simulink model "HighFiedelity_Simulation"  (R2021b)
settings: Solver=ode45  StartTime=0  StopTime=Stop_Time  FixedStep=Simstep  MaxStep=Simstep  RelTol=1e-5  EnableMultiTasking=on
values from neighbouring files (symbols this model uses):
  Angle_idx = linspace(0,Angle_max,Angle_step)    [A_ToyotaPrius_Flux_Model_Parameter.m]    (also in B1_IPMSM_Machine_Parameter_Init.m)
  Angle_idx_initial = (length(Angle_idx)+1)/2    [A_ToyotaPrius_Flux_Model_Parameter.m]    (also in B1_IPMSM_Machine_Parameter_Init.m)
  flux_d_idx = ParamFluxDIndex    [A_ToyotaPrius_Flux_Model_Parameter.m]    (also in B1_IPMSM_Machine_Parameter_Init.m)
  flux_q_idx = ParamFluxQIndex    [A_ToyotaPrius_Flux_Model_Parameter.m]    (also in B1_IPMSM_Machine_Parameter_Init.m)
  FluxD_Id_Iq_Theta = reshape(Flux_d,Angle_step,I_step,I_step)    [A_ToyotaPrius_Flux_Model_Parameter.m]    (also in B1_IPMSM_Machine_Parameter_Init.m)
  FluxQ_Id_Iq_Theta = reshape(Flux_q,Angle_step,I_step,I_step)    [A_ToyotaPrius_Flux_Model_Parameter.m]    (also in B1_IPMSM_Machine_Parameter_Init.m)
  I_step = 21    [A_ToyotaPrius_Flux_Model_Parameter.m]    (also in B1_IPMSM_Machine_Parameter_Init.m)
  Id_idx = linspace(I_min,I_max,I_step)    [A_ToyotaPrius_Flux_Model_Parameter.m]    (also in B1_IPMSM_Machine_Parameter_Init.m)
  Iq_idx = linspace(I_min,I_max,I_step)    [A_ToyotaPrius_Flux_Model_Parameter.m]    (also in B1_IPMSM_Machine_Parameter_Init.m)
  Step_Time = [0 1 2 3 4 5]    [A0_HighFidelitySimulation.m]    (also in B_PMSM.m = [0.25 0.5 0.75 1])
  Te_Ref_Set = [0.0001 0.00001 0.2 0.3 0.4 0.5]*Motor1.Te_Rated    [A0_HighFidelitySimulation.m]    (also in B_PMSM.m = ones(1,5)*Te_Rated*1)
  Te_SlewRate = inf    [A0_HighFidelitySimulation.m]    (also in B_PMSM.m)
  Torque_Id_Iq_Theta = reshape(Torque_e,Angle_step,I_step,I_step)    [A_ToyotaPrius_Flux_Model_Parameter.m]    (also in B1_IPMSM_Machine_Parameter_Init.m)
  TrqIdmap = ATICALParameterList.Table3D(1).ZAxis    [A_ToyotaPrius_Flux_Model_Parameter.m]    (also in C1_INV1_GainSetting.m)
  TrqIqmap = ATICALParameterList.Table3D(2).ZAxis    [A_ToyotaPrius_Flux_Model_Parameter.m]    (also in C1_INV1_GainSetting.m)
  TrqTId = ATICALParameterList.Table3D(1).YAxis    [A_ToyotaPrius_Flux_Model_Parameter.m]    (also in C1_INV1_GainSetting.m)
  TrqTIq = ATICALParameterList.Table3D(2).YAxis    [A_ToyotaPrius_Flux_Model_Parameter.m]    (also in C1_INV1_GainSetting.m)
  TrqWrId = ATICALParameterList.Table3D(1).XAxis    [A_ToyotaPrius_Flux_Model_Parameter.m]    (also in C1_INV1_GainSetting.m)
  TrqWrIq = ATICALParameterList.Table3D(2).XAxis    [A_ToyotaPrius_Flux_Model_Parameter.m]    (also in C1_INV1_GainSetting.m)
  Vdc = 650    [A0_HighFidelitySimulation.m]    (also in B_PMSM.m)
  Wrpm_Ref_Set = [5000 5000 5000 5000 5000]    [A0_HighFidelitySimulation.m]    (also in B_PMSM.m = Wrm_Init*ones(1,5))
undefined symbols (not defined in the file or in its folder): DCMotor, DiscIntNeverNeededParam, idmap, INV1, INV2, iqmap, Motor1
libraries: simulink x3
settings Model: SimulationMode=accelerator  Creator=KYC  LastModifiedBy=jun
settings SolverCC: AlgebraicLoopSolver=TrustRegion
settings DataIOCC: LimitDataPoints=on  SaveFormat=Array  ReturnWorkspaceOutputs=off
settings OptimizationCC: LifeSpan=inf
settings DebuggingCC: UnderspecifiedInitializationDetection=Classic  MergeDetectMultiDrivingBlocksExec=none  SolverPrmCheckMsg=warning  InheritedTsInSrcMsg=none  AllowSymbolicDim=off  StateNameClashWarn=warning  SFUnexpectedBacktrackingDiag=warning  SFNoUnconditionalDefaultTransitionDiag=warning  SFExecutionAtInitializationDiag=none  SFMachineParentedDataDiag=warning  ArithmeticOperatorsInVariantConditions=warning
settings HardwareCC: ProdBitPerPointer=32  ProdBitPerSizeT=32  ProdBitPerPtrDiffT=32  ProdLargestAtomicFloat=None  ProdIntDivRoundTo=Undefined  ProdEndianess=Unspecified  ProdWordSize=32  ProdHWDeviceType=32-bit Generic
settings ModelReferenceCC: PropagateSignalLabelsOutOfModel=off
settings SFSimCC: SimUseLocalCustomCode=off  CustomCodeUndefinedFunction=UseInterfaceOnly
settings RTWCC: RTWUseLocalCustomCode=off
settings CodeAppCC: StateflowObjectComments=on
settings GRTTargetCC: TargetLangStandard=C89/C90 (ANSI)
settings ConfigComp: CovMetricSettings=dw  CovSaveCumulativeToWorkspaceVar=on  CovSaveSingleToWorkspaceVar=on  CovExternalEMLEnable=off  CovSFcnEnable=off

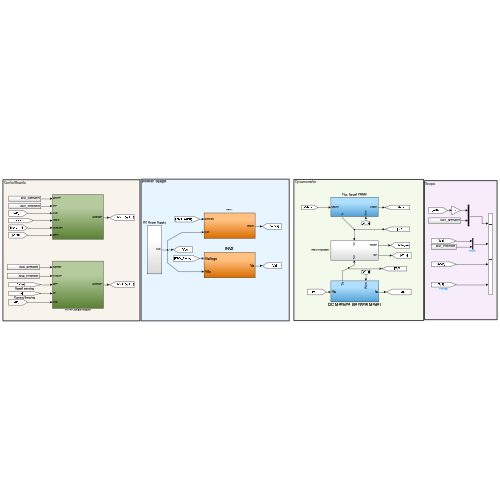
[thumbnail: Simulink's stored preview of the top-level diagram]
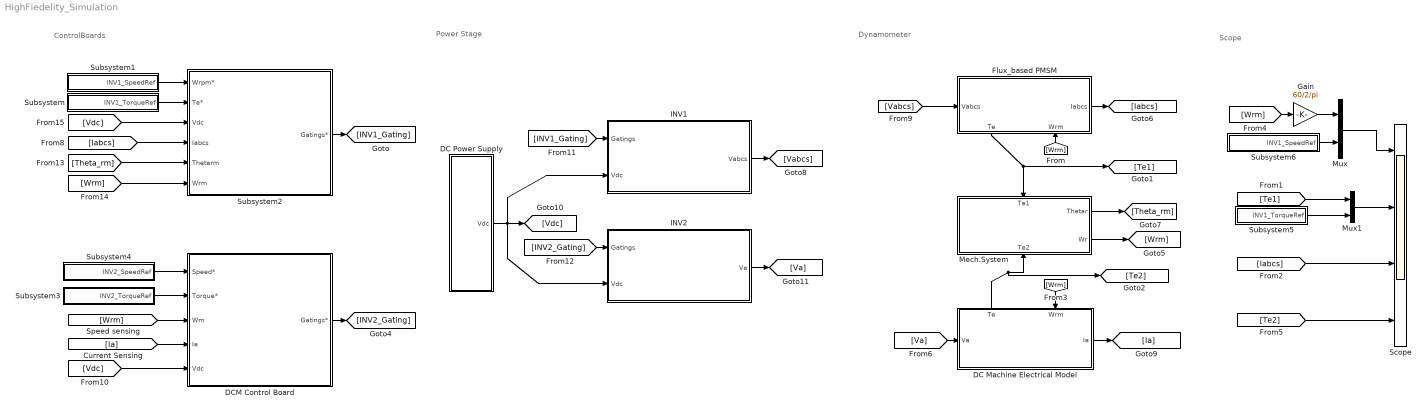
== system HighFiedelity_Simulation ==
  note: Scope
  note: ControlBoards
  note: Dynamometer
  note: Power Stage
  DC Machine Electrical Model : Subsystem
      settings: PortSchema="{\"entries\":[{\"content\":{\"sides\":[{\"content\":{\"connectorIds\":[\"In1\"]},\"type\":\"ConnectorPlacement.EquallySpacedRectSide\",\"uuid\":\"4074897e-6920-4f33-b302-64d86120b7df\"},{\"content\":{\"connectorIds\":[\"Out1\"],\"side\":\"RIGHT\"},\"type\":\"ConnectorPlacement.EquallySpacedRectSide\",\"uuid\":\"671615ca-e362-48c9-a030-03d33faae874\"},{\"content\":{\"connectorIds\":[\"Out2\",\"In2\"],\"side\":\"TOP\"},\"type\":\"ConnectorPlacement.EquallySpacedRectSide\",\"uuid\":\"d587e8fb-b462-47db-b9f9-66f25c83a3fe\"},{\"content\":{\"connectorIds\":[],\"side\":\"BOTTOM\"},\"type\":\"ConnectorPlacement.EquallySpacedRectSide\",\"uuid\":\"9be21003-cb0d-41fd-b790-e70774da76cb\"}]},\"type\":\"ConnectorPlacement.EquallySpacedConnector\",\"uuid\":\"22d4a5b5-b610-40ac-ac45-102e1f1adc00\"}],\"packageUris\":[\"http://schema.mathworks.com/mf0/Connector/R2020b\"],\"version\":\"1.0\"}"
  DC Power Supply : Subsystem
  DCM Control Board : Subsystem
  Flux_based PMSM : Subsystem
      settings: PortSchema="{\"entries\":[{\"content\":{\"sides\":[{\"content\":{\"connectorIds\":[\"In1\"]},\"type\":\"ConnectorPlacement.EquallySpacedRectSide\",\"uuid\":\"24322e7c-2896-443d-bb86-37c4d4149ef5\"},{\"content\":{\"connectorIds\":[\"Out1\"],\"side\":\"RIGHT\"},\"type\":\"ConnectorPlacement.EquallySpacedRectSide\",\"uuid\":\"a5d08852-92bf-4b5a-af83-42822b482983\"},{\"content\":{\"connectorIds\":[],\"side\":\"TOP\"},\"type\":\"ConnectorPlacement.EquallySpacedRectSide\",\"uuid\":\"64930a76-1018-4eab-af8e-9c2112ff20c6\"},{\"content\":{\"connectorIds\":[\"Out2\",\"In2\"],\"side\":\"BOTTOM\"},\"type\":\"ConnectorPlacement.EquallySpacedRectSide\",\"uuid\":\"89450d1c-3f7d-44a3-8810-d67b8ce20cc5\"}]},\"type\":\"ConnectorPlacement.EquallySpacedConnector\",\"uuid\":\"0cf1f8cb-98d5-4acc-99e3-a93106a75429\"}],\"packageUris\":[\"http://schema.mathworks.com/mf0/Connector/R2020b\"],\"version\":\"1.0\"}"
  Gain : Gain  Gain=60/2/pi
  INV1 : Subsystem
  INV2 : Subsystem
  Mech.System : Subsystem
      settings: PortSchema="{\"entries\":[{\"content\":{\"sides\":[{\"content\":{\"connectorIds\":[]},\"type\":\"ConnectorPlacement.EquallySpacedRectSide\",\"uuid\":\"7816393c-e6ef-44df-b641-25156ded1cdc\"},{\"content\":{\"connectorIds\":[\"Out1\",\"Out2\"],\"side\":\"RIGHT\"},\"type\":\"ConnectorPlacement.EquallySpacedRectSide\",\"uuid\":\"df3d9513-253d-4c97-8efd-af2438fb286e\"},{\"content\":{\"connectorIds\":[\"In1\"],\"side\":\"TOP\"},\"type\":\"ConnectorPlacement.EquallySpacedRectSide\",\"uuid\":\"65b6b526-a008-40f6-a42d-b2e1dc0c5f24\"},{\"content\":{\"connectorIds\":[\"In2\"],\"side\":\"BOTTOM\"},\"type\":\"ConnectorPlacement.EquallySpacedRectSide\",\"uuid\":\"f448aff5-19c1-43a0-84ba-52356c379f88\"}]},\"type\":\"ConnectorPlacement.EquallySpacedConnector\",\"uuid\":\"afd6e091-39ce-476c-80f4-568492feeb85\"}],\"packageUris\":[\"http://schema.mathworks.com/mf0/Connector/R2020b\"],\"version\":\"1.0\"}"
  Mux : Mux  Inputs=2
  Mux1 : Mux  Inputs=2
  Scope : Scope  NumInputPorts=4
  Subsystem : Subsystem
  Subsystem1 : Subsystem
  Subsystem2 : Subsystem
  Subsystem3 : Subsystem
  Subsystem4 : Subsystem
  Subsystem5 : Subsystem
  Subsystem6 : Subsystem
  wires:
  Flux_based PMSM/1(Iabcs) -> [Iabcs]
  [Vabcs] -> Flux_based PMSM/1(Vabcs)
  DCM Control Board/1(Gatings*) -> [INV2_Gating]
  [Wrm] -> DCM Control Board/3(Wm)
  [Vdc] -> DCM Control Board/5(Vdc)
  [Ia] -> DCM Control Board/4(Ia)
  Subsystem3/1(INV2_TorqueRef) -> DCM Control Board/2(Torque*)
  Mech.System/2(Wr) -> [Wrm]
  Mech.System/1(Thetar) -> [Theta_rm]
  DC Machine Electrical Model/2(Te) -> [Te2], Mech.System/2(Te2)
  Flux_based PMSM/2(Te) -> [Te1], Mech.System/1(Te1)
  [INV1_Gating] -> INV1/1(Gatings)
  [INV2_Gating] -> INV2/1(Gatings)
  DC Power Supply/1(Vdc) -> INV1/2(Vdc), [Vdc], INV2/2(Vdc)
  INV1/1(Vabcs) -> [Vabcs]
  INV2/1(Va) -> [Va]
  Subsystem2/1(Gatings*) -> [INV1_Gating]
  [Wrm] -> Flux_based PMSM/2(Wrm)
  [Wrm] -> DC Machine Electrical Model/2(Wrm)
  [Va] -> DC Machine Electrical Model/1(Va)
  Subsystem1/1(INV1_SpeedRef) -> Subsystem2/1(Wrpm*)
  Subsystem/1(INV1_TorqueRef) -> Subsystem2/2(Te*)
  [Vdc] -> Subsystem2/3(Vdc)
  [Iabcs] -> Subsystem2/4(Iabcs)
  [Theta_rm] -> Subsystem2/5(Thetarm)
  [Wrm] -> Subsystem2/6(Wrm)
  [Wrm] -> Gain/1
  Gain/1 -> Mux/1
  Subsystem6/1(INV1_SpeedRef) -> Mux/2
  Mux/1 -> Scope/1
  [Iabcs] -> Scope/3
  Subsystem5/1(INV1_TorqueRef) -> Mux1/2
  Mux1/1 -> Scope/2
  [Te1] -> Mux1/1
  DC Machine Electrical Model/1(Ia) -> [Ia]
  Subsystem4/1(INV2_SpeedRef) -> DCM Control Board/1(Speed*)
  [Te2] -> Scope/4

== system HighFiedelity_Simulation/DC Machine Electrical Model ==
  note: DC Machine Electrical Model
  Va : Inport
  Wrm : Inport  Port=2
  1/La2 : Gain  Gain=DCMotor.K  SaturateOnIntegerOverflow=on  OutDataTypeStr=Inherit: Same as input  ParamDataTypeStr=Inherit: Same as input
  Gain2 : Gain  Gain=1/DCMotor.La
  Gain3 : Gain  Gain=DCMotor.Ra
  Gain4 : Gain  Gain=DCMotor.K
  Integrator1 : Integrator
  Sum : Sum  Inputs=+--  SaturateOnIntegerOverflow=on
  Ia : Outport
  Te : Outport  Port=2  VectorParamsAs1DForOutWhenUnconnected=off
  wires:
  1/La2/1 -> Sum/2
  Integrator1/1 -> Gain4/1, Ia/1, Gain3/1
  Sum/1 -> Gain2/1
  Gain4/1 -> Te/1
  Va/1 -> Sum/1
  Gain2/1 -> Integrator1/1
  Gain3/1 -> Sum/3
  Wrm/1 -> 1/La2/1

== system HighFiedelity_Simulation/DC Power Supply ==
  Constant : Constant  Value=Vdc
  Vdc : Outport
  wires:
  Constant/1 -> Vdc/1

== system HighFiedelity_Simulation/DCM Control Board ==
  Speed* : Inport
  Torque* : Inport  Port=2
  Wm : Inport  Port=3
  Ia : Inport  Port=4
  Vdc : Inport  Port=5
  Control Programs : Subsystem
  Fsw : DiscretePulseGenerator  PulseType=Time based  Period=1/INV2.SwitchingFrequency  PulseWidth=50
  Gain : Gain  Gain=-1
  PWM Module : Subsystem
  Gatings* : Outport
  wires:
  PWM Module/1(Gating) -> Gatings*/1
  Speed*/1 -> Control Programs/1(Speed*)
  Torque*/1 -> Control Programs/2(Torque*)
  Wm/1 -> Gain/1
  Ia/1 -> Control Programs/4(Ia)
  Fsw/1 -> Control Programs/Trigger
  Control Programs/1(Counter) -> PWM Module/1(Counter)
  Vdc/1 -> Control Programs/5(Vdc)
  Gain/1 -> Control Programs/3(Wm)

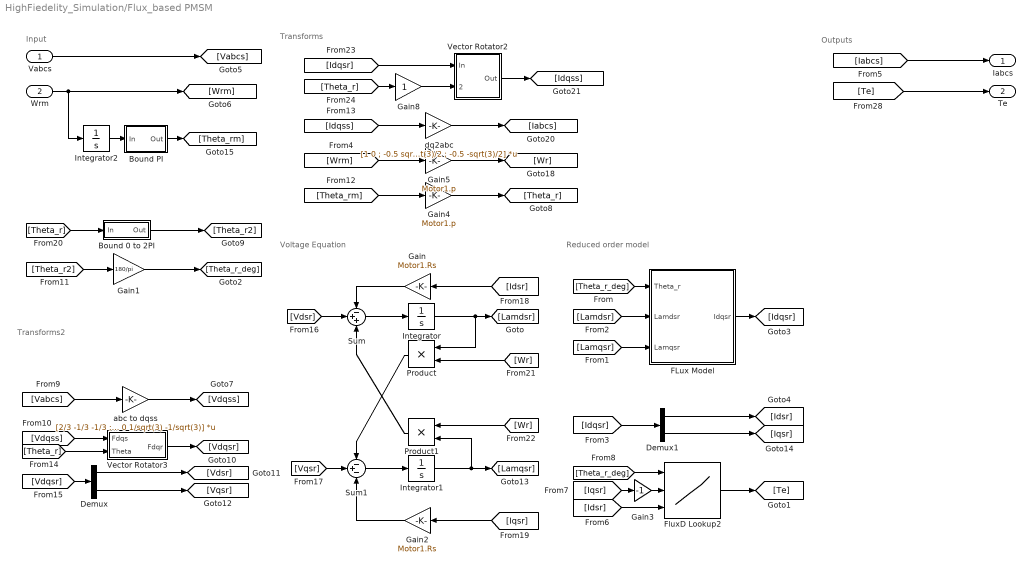
== system HighFiedelity_Simulation/Flux_based PMSM ==
  note: Transforms
  note: Reduced order model
  note: Voltage Equation
  note: Transforms2
  note: Input
  note: Outputs
  Vabcs : Inport
  Wrm : Inport  Port=2
  Bound 0 to 2PI : Subsystem
  Bound PI : Subsystem
  Demux : Demux  Outputs=2
  Demux1 : Demux  Outputs=2
  FLux Model : Subsystem
  FluxD Lookup2 : Lookup_n-D  NumberOfTableDimensions=3  BreakpointsForDimension1=Angle_idx  BreakpointsForDimension2=Id_idx  BreakpointsForDimension3=Iq_idx  Table=Torque_Id_Iq_Theta  InternalRulePriority=Speed  RndMeth=Simplest  InputSameDT=on
      settings: InputPortMap=u0,u1,u2
  Gain : Gain  Gain=Motor1.Rs
  Gain1 : Gain  Gain=180/pi
  Gain2 : Gain  Gain=Motor1.Rs
  Gain3 : Gain  Gain=-1
  Gain4 : Gain  Gain=Motor1.p
  Gain5 : Gain  Gain=Motor1.p
  Gain8 : Gain
  Integrator : Integrator  InitialCondition=FluxD_Id_Iq_Theta(Angle_idx_initial,(I_step+1)/2,(I_step+1)/2)
  Integrator1 : Integrator  InitialCondition=FluxQ_Id_Iq_Theta(Angle_idx_initial,(I_step+1)/2,(I_step+1)/2)
  Integrator2 : Integrator
  Product : Product
  Product1 : Product
  Sum : Sum  Inputs=-++
  Sum1 : Sum  Inputs=-+-
  Vector Rotator2 : Subsystem
  Vector Rotator3 : Subsystem
  abc to dqss : Gain  Gain=[2/3 -1/3 -1/3 ; 0 1/sqrt(3) -1/sqrt(3)]  Multiplication=Matrix(K*u)
  dq2abc : Gain  Gain=[1 0 ; -0.5 sqrt(3)/2 ; -0.5 -sqrt(3)/2]  Multiplication=Matrix(K*u)
  Iabcs : Outport
  Te : Outport  Port=2
  wires:
  [Theta_r] -> Vector Rotator3/2(Theta)
  Vabcs/1 -> [Vabcs]
  [Vdqss] -> Vector Rotator3/1(Fdqs)
  Vector Rotator3/1(Fdqr) -> [Vdqsr]
  [Vabcs] -> abc to dqss/1
  abc to dqss/1 -> [Vdqss]
  Bound 0 to 2PI/1(Out) -> [Theta_r2]
  [Theta_r] -> Bound 0 to 2PI/1(In)
  [Theta_r2] -> Gain1/1
  [Iqsr] -> Gain3/1
  [Idsr] -> FluxD Lookup2/3
  [Theta_r_deg] -> FluxD Lookup2/1
  [Vdqsr] -> Demux/1
  Demux/2 -> [Vqsr]
  Demux/1 -> [Vdsr]
  [Vdsr] -> Sum/2
  [Vqsr] -> Sum1/2
  Gain/1 -> Sum/1
  [Idsr] -> Gain/1
  [Iqsr] -> Gain2/1
  Gain2/1 -> Sum1/3
  Sum/1 -> Integrator/1
  Integrator/1 -> Product/1, [Lamdsr]
  [Wr] -> Product/2
  Product/1 -> Sum1/1
  Sum1/1 -> Integrator1/1
  Integrator1/1 -> Product1/2, [Lamqsr]
  [Wr] -> Product1/1
  Product1/1 -> Sum/3
  [Theta_r_deg] -> FLux Model/1(Theta_r)
  [Lamdsr] -> FLux Model/2(Lamdsr)
  [Lamqsr] -> FLux Model/3(Lamqsr)
  [Idqsr] -> Demux1/1
  Demux1/2 -> [Iqsr]
  Gain1/1 -> [Theta_r_deg]
  Gain3/1 -> FluxD Lookup2/2
  FLux Model/1(Idqsr) -> [Idqsr]
  Gain4/1 -> [Theta_r]
  [Idqss] -> dq2abc/1
  dq2abc/1 -> [Iabcs]
  Gain5/1 -> [Wr]
  [Wrm] -> Gain5/1
  [Theta_rm] -> Gain4/1
  Vector Rotator2/1(Out) -> [Idqss]
  [Theta_r] -> Gain8/1
  Gain8/1 -> Vector Rotator2/2(Theta)
  [Idqsr] -> Vector Rotator2/1(In)
  [Iabcs] -> Iabcs/1
  [Te] -> Te/1
  FluxD Lookup2/1 -> [Te]
  Demux1/1 -> [Idsr]
  Wrm/1 -> Integrator2/1, [Wrm]
  Bound PI/1(Out) -> [Theta_rm]
  Integrator2/1 -> Bound PI/1(In)

== system HighFiedelity_Simulation/INV1 ==
  Gatings : Inport
  Vdc : Inport  Port=2
  Product : Product
  Vabcs : Outport
  wires:
  Gatings/1 -> Product/1
  Vdc/1 -> Product/2
  Product/1 -> Vabcs/1

== system HighFiedelity_Simulation/INV2 ==
  Gatings : Inport
  Vdc : Inport  Port=2
  Product : Product
  Va : Outport  InitialOutput=0  VectorParamsAs1DForOutWhenUnconnected=off
  wires:
  Vdc/1 -> Product/2
  Product/1 -> Va/1
  Gatings/1 -> Product/1

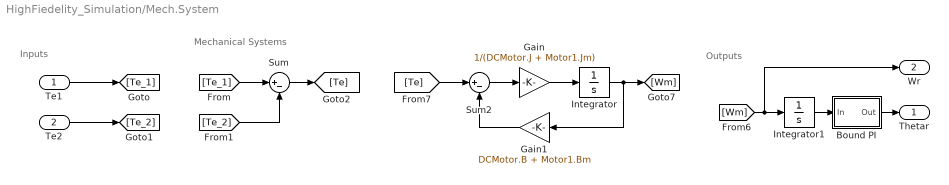
== system HighFiedelity_Simulation/Mech.System ==
  note: Outputs
  note: Mechanical Systems
  note: Inputs
  Te1 : Inport
  Te2 : Inport  Port=2
  Bound PI : Subsystem
  Gain : Gain  Gain=1/(DCMotor.J + Motor1.Jm)
  Gain1 : Gain  Gain=DCMotor.B + Motor1.Bm
  Integrator : Integrator
  Integrator1 : Integrator
  Sum : Sum  Inputs=|+-
  Sum2 : Sum  Inputs=|+-
  Thetar : Outport  VectorParamsAs1DForOutWhenUnconnected=off
  Wr : Outport  Port=2
  wires:
  Sum2/1 -> Gain/1
  Gain1/1 -> Sum2/2
  Gain/1 -> Integrator/1
  Integrator/1 -> Gain1/1, [Wm]
  Te1/1 -> [Te_1]
  Te2/1 -> [Te_2]
  [Te_1] -> Sum/1
  [Te_2] -> Sum/2
  Sum/1 -> [Te]
  [Te] -> Sum2/1
  Bound PI/1(Out) -> Thetar/1
  Integrator1/1 -> Bound PI/1(In)
  [Wm] -> Wr/1, Integrator1/1

== system HighFiedelity_Simulation/Subsystem ==
  Add : Sum  Inputs=++++
  Rate Limiter : RateLimiter  RisingSlewLimit=Te_SlewRate*Motor1.Te_Rated  FallingSlewLimit=-Te_SlewRate*Motor1.Te_Rated  SampleTimeMode=inherited
  Scope : Scope  NumInputPorts=2
  Step1 : Step  Time=Step_Time(1)  Before=Te_Ref_Set(1)  After=Te_Ref_Set(2)
  Step2 : Step  Time=Step_Time(3)  After=Te_Ref_Set(4)-Te_Ref_Set(3)
  Step3 : Step  Time=Step_Time(2)  After=Te_Ref_Set(3)-Te_Ref_Set(2)
  Step4 : Step  Time=Step_Time(4)  After=Te_Ref_Set(5)-Te_Ref_Set(4)
  INV1_TorqueRef : Outport
  wires:
  Step2/1 -> Add/3
  Step4/1 -> Add/4
  Step3/1 -> Add/2
  Step1/1 -> Add/1
  Rate Limiter/1 -> Scope/2, INV1_TorqueRef/1
  Add/1 -> Scope/1, Rate Limiter/1

== system HighFiedelity_Simulation/Subsystem1 ==
  Add : Sum  Inputs=++++
  Step1 : Step  Time=Step_Time(1)  Before=Wrpm_Ref_Set(1)  After=Wrpm_Ref_Set(2)
  Step2 : Step  Time=Step_Time(3)  After=Wrpm_Ref_Set(4)-Wrpm_Ref_Set(3)
  Step3 : Step  Time=Step_Time(2)  After=Wrpm_Ref_Set(3)-Wrpm_Ref_Set(2)
  Step4 : Step  Time=Step_Time(4)  After=Wrpm_Ref_Set(5)-Wrpm_Ref_Set(4)
  INV1_SpeedRef : Outport
  wires:
  Step1/1 -> Add/1
  Step3/1 -> Add/2
  Step4/1 -> Add/4
  Step2/1 -> Add/3
  Add/1 -> INV1_SpeedRef/1

== system HighFiedelity_Simulation/Subsystem2 ==
  Wrpm* : Inport
  Te* : Inport  Port=2
  Vdc : Inport  Port=3
  Iabcs : Inport  Port=4
  Thetarm : Inport  Port=5
  Wrm : Inport  Port=6
  Digital Controller : Subsystem
  PWM Module : Subsystem
  Pulse Generator2 : DiscretePulseGenerator  PulseType=Time based  Period=INV1.Ts  PulseWidth=50
  Gatings* : Outport
  wires:
  Digital Controller/1(Counter) -> PWM Module/1(Counter)
  Iabcs/1 -> Digital Controller/4(Iabcs)
  Te*/1 -> Digital Controller/2(Te*)
  Thetarm/1 -> Digital Controller/5(Thetarm)
  Pulse Generator2/1 -> Digital Controller/Trigger
  Vdc/1 -> Digital Controller/3(Vdc)
  Wrm/1 -> Digital Controller/6(Wrm)
  Wrpm*/1 -> Digital Controller/1(Wrpm*)
  PWM Module/1(Gatings) -> Gatings*/1

== system HighFiedelity_Simulation/Subsystem3 ==
  Add : Sum  Inputs=++++
  Rate Limiter : RateLimiter  RisingSlewLimit=Te_SlewRate*Motor1.Te_Rated  FallingSlewLimit=-Te_SlewRate*Motor1.Te_Rated  SampleTimeMode=inherited
  Step1 : Step  Time=Step_Time(1)  Before=Te_Ref_Set(1)  After=Te_Ref_Set(2)
  Step2 : Step  Time=Step_Time(3)  After=Te_Ref_Set(4)-Te_Ref_Set(3)
  Step3 : Step  Time=Step_Time(2)  After=Te_Ref_Set(3)-Te_Ref_Set(2)
  Step4 : Step  Time=Step_Time(4)  After=Te_Ref_Set(5)-Te_Ref_Set(4)
  INV2_TorqueRef : Outport
  wires:
  Step2/1 -> Add/3
  Step4/1 -> Add/4
  Step3/1 -> Add/2
  Step1/1 -> Add/1
  Rate Limiter/1 -> INV2_TorqueRef/1
  Add/1 -> Rate Limiter/1

== system HighFiedelity_Simulation/Subsystem4 ==
  Add : Sum  Inputs=++++
  Gain : Gain  Gain=-1
  Step1 : Step  Time=Step_Time(1)  Before=Wrpm_Ref_Set(1)  After=Wrpm_Ref_Set(2)
  Step2 : Step  Time=Step_Time(3)  After=Wrpm_Ref_Set(4)-Wrpm_Ref_Set(3)
  Step3 : Step  Time=Step_Time(2)  After=Wrpm_Ref_Set(3)-Wrpm_Ref_Set(2)
  Step4 : Step  Time=Step_Time(4)  After=Wrpm_Ref_Set(5)-Wrpm_Ref_Set(4)
  INV2_SpeedRef : Outport
  wires:
  Step1/1 -> Add/1
  Step3/1 -> Add/2
  Step4/1 -> Add/4
  Step2/1 -> Add/3
  Gain/1 -> INV2_SpeedRef/1
  Add/1 -> Gain/1

== system HighFiedelity_Simulation/Subsystem5 ==
  Add : Sum  Inputs=++++
  Rate Limiter : RateLimiter  RisingSlewLimit=Te_SlewRate*Motor1.Te_Rated  FallingSlewLimit=-Te_SlewRate*Motor1.Te_Rated  SampleTimeMode=inherited
  Step1 : Step  Time=Step_Time(1)  Before=Te_Ref_Set(1)  After=Te_Ref_Set(2)
  Step2 : Step  Time=Step_Time(3)  After=Te_Ref_Set(4)-Te_Ref_Set(3)
  Step3 : Step  Time=Step_Time(2)  After=Te_Ref_Set(3)-Te_Ref_Set(2)
  Step4 : Step  Time=Step_Time(4)  After=Te_Ref_Set(5)-Te_Ref_Set(4)
  INV1_TorqueRef : Outport
  wires:
  Step2/1 -> Add/3
  Step4/1 -> Add/4
  Step3/1 -> Add/2
  Step1/1 -> Add/1
  Rate Limiter/1 -> INV1_TorqueRef/1
  Add/1 -> Rate Limiter/1

== system HighFiedelity_Simulation/Subsystem6 ==
  Add : Sum  Inputs=++++
  Step1 : Step  Time=Step_Time(1)  Before=Wrpm_Ref_Set(1)  After=Wrpm_Ref_Set(2)
  Step2 : Step  Time=Step_Time(3)  After=Wrpm_Ref_Set(4)-Wrpm_Ref_Set(3)
  Step3 : Step  Time=Step_Time(2)  After=Wrpm_Ref_Set(3)-Wrpm_Ref_Set(2)
  Step4 : Step  Time=Step_Time(4)  After=Wrpm_Ref_Set(5)-Wrpm_Ref_Set(4)
  INV1_SpeedRef : Outport
  wires:
  Step1/1 -> Add/1
  Step3/1 -> Add/2
  Step4/1 -> Add/4
  Step2/1 -> Add/3
  Add/1 -> INV1_SpeedRef/1

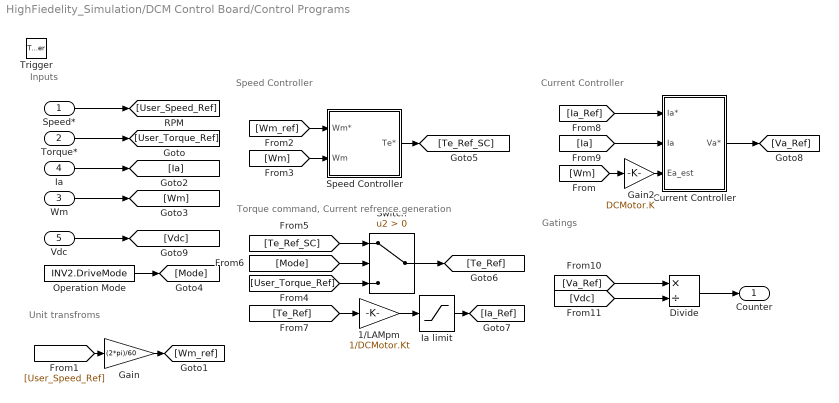
== system HighFiedelity_Simulation/DCM Control Board/Control Programs ==
  note: Speed Controller
  note: Unit transfroms
  note: Inputs
  note: Current Controller
  note: Gatings
  note: Torque command, Current refrence generation
  Speed* : Inport
  Torque* : Inport  Port=2
  Wm : Inport  Port=3
  Ia : Inport  Port=4
  Vdc : Inport  Port=5
  Trigger : TriggerPort  VariantControl=(inherit)  PortDimensions=1
  1/LAMpm : Gain  Gain=1/DCMotor.Kt  SaturateOnIntegerOverflow=on  OutDataTypeStr=Inherit: Same as input  ParamDataTypeStr=Inherit: Same as input
  Current Controller : Subsystem
  Divide : Product  Inputs=*/
  Gain : Gain  Gain=(2*pi)/60
  Gain2 : Gain  Gain=DCMotor.K
  Ia limit : Saturate  UpperLimit=DCMotor.Ia_limit  LowerLimit=-DCMotor.Ia_limit
  Operation Mode : Constant  Value=INV2.DriveMode
  Speed Controller : Subsystem
  Switch : Switch  Criteria=u2 > Threshold
  Counter : Outport
  wires:
  Speed*/1 -> [User_Speed_Ref]
  Gain/1 -> [Wm_ref]
  Gain2/1 -> Current Controller/3(Ea_est)
  Torque*/1 -> [User_Torque_Ref]
  [Te_Ref] -> 1/LAMpm/1
  Speed Controller/1(Te*) -> [Te_Ref_SC]
  Ia/1 -> [Ia]
  [Ia_Ref] -> Current Controller/1(Ia*)
  Switch/1 -> [Te_Ref]
  [Ia] -> Current Controller/2(Ia)
  [Mode] -> Switch/2
  Ia limit/1 -> [Ia_Ref]
  Operation Mode/1 -> [Mode]
  [User_Torque_Ref] -> Switch/3
  [Wm] -> Gain2/1
  1/LAMpm/1 -> Ia limit/1
  [User_Speed_Ref] -> Gain/1
  [Te_Ref_SC] -> Switch/1
  [Wm] -> Speed Controller/2(Wm)
  [Wm_ref] -> Speed Controller/1(Wm*)
  Wm/1 -> [Wm]
  Vdc/1 -> [Vdc]
  [Va_Ref] -> Divide/1
  Divide/1 -> Counter/1
  [Vdc] -> Divide/2
  Current Controller/1(Va*) -> [Va_Ref]

== system HighFiedelity_Simulation/DCM Control Board/PWM Module ==
  Counter : Inport
  Carrier wave : simulink/Sources/Repeating Sequence  rep_seq_t="[0  1/2/INV2.SwitchingFrequency  1/INV2.SwitchingFrequency]"  rep_seq_y=[-1 1 -1]
  Sum2 : Sum  Inputs=+-  SaturateOnIntegerOverflow=on
  Gating : Outport
  wires:
  Counter/1 -> Sum2/1
  Carrier wave/1 -> Sum2/2
  Sum2/1 -> Gating/1

== system HighFiedelity_Simulation/Flux_based PMSM/Bound 0 to 2PI ==
  In : Inport
  Fcn1 : Fcn  Expr=1/(2*pi)*u+0.5
  Fcn2 : Fcn  Expr=u-floor(u)
  Fcn3 : Fcn  Expr=2*pi*(u)
  Out : Outport
  wires:
  Fcn1/1 -> Fcn2/1
  Fcn2/1 -> Fcn3/1
  In/1 -> Fcn1/1
  Fcn3/1 -> Out/1

== system HighFiedelity_Simulation/Flux_based PMSM/Bound PI ==
  In : Inport
  Fcn1 : Fcn  Expr=1/(2*pi)*u+0.5
  Fcn2 : Fcn  Expr=u-floor(u)
  Fcn3 : Fcn  Expr=2*pi*(u-0.5)
  Out : Outport
  wires:
  Fcn1/1 -> Fcn2/1
  Fcn2/1 -> Fcn3/1
  In/1 -> Fcn1/1
  Fcn3/1 -> Out/1

== system HighFiedelity_Simulation/Flux_based PMSM/FLux Model ==
  Theta_r : Inport
  Lamdsr : Inport  Port=2
  Lamqsr : Inport  Port=3
  IC : InitialCondition  Value=0
  IC1 : InitialCondition  Value=0
  Id Lookup : Lookup_n-D  NumberOfTableDimensions=3  BreakpointsForDimension1=Angle_idx  BreakpointsForDimension2=flux_d_idx  BreakpointsForDimension3=flux_q_idx  Table=idmap  InternalRulePriority=Speed  RndMeth=Simplest  InputSameDT=on
      settings: InputPortMap=u0,u1,u2
  Iq Lookup : Lookup_n-D  NumberOfTableDimensions=3  BreakpointsForDimension1=Angle_idx  BreakpointsForDimension2=flux_d_idx  BreakpointsForDimension3=flux_q_idx  Table=iqmap  InternalRulePriority=Speed  RndMeth=Simplest  InputSameDT=on
      settings: InputPortMap=u0,u1,u2
  Mux : Mux  Inputs=2
  Idqsr : Outport
  wires:
  Iq Lookup/1 -> IC1/1
  Theta_r/1 -> Iq Lookup/1, Id Lookup/1
  Id Lookup/1 -> IC/1
  Mux/1 -> Idqsr/1
  IC/1 -> Mux/1
  IC1/1 -> Mux/2
  Lamqsr/1 -> Id Lookup/3, Iq Lookup/3
  Lamdsr/1 -> Iq Lookup/2, Id Lookup/2

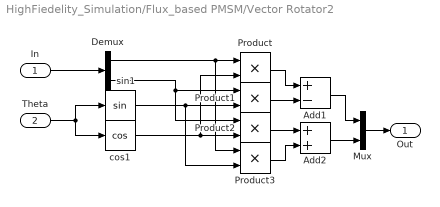
== system HighFiedelity_Simulation/Flux_based PMSM/Vector Rotator2 ==
  In : Inport
  Theta : Inport  Port=2
  Add1 : Sum  Inputs=+-
  Add2 : Sum
  Demux : Demux  Outputs=2
  Mux : Mux  Inputs=[1 1]
  Product{,1..3} (4 alike) : Product  RndMeth=Zero
  cos1 : Trigonometry  Operator=cos
  sin1 : Trigonometry
  Out : Outport
  wires:
  Theta/1 -> cos1/1, sin1/1
  Demux/1 -> Product3/1, Product/1
  Mux/1 -> Out/1
  In/1 -> Demux/1
  Demux/2 -> Product1/1, Product2/1
  cos1/1 -> Product/2, Product2/2
  sin1/1 -> Product1/2, Product3/2
  Product/1 -> Add1/1
  Product1/1 -> Add1/2
  Add1/1 -> Mux/1
  Product2/1 -> Add2/1
  Product3/1 -> Add2/2
  Add2/1 -> Mux/2

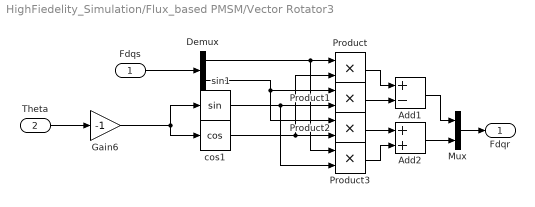
== system HighFiedelity_Simulation/Flux_based PMSM/Vector Rotator3 ==
  Fdqs : Inport
  Theta : Inport  Port=2
  Add1 : Sum  Inputs=+-
  Add2 : Sum
  Demux : Demux  Outputs=2
  Gain6 : Gain  Gain=-1
  Mux : Mux  Inputs=[1 1]
  Product{,1..3} (4 alike) : Product  RndMeth=Zero
  cos1 : Trigonometry  Operator=cos
  sin1 : Trigonometry
  Fdqr : Outport
  wires:
  Theta/1 -> Gain6/1
  Demux/1 -> Product3/1, Product/1
  Mux/1 -> Fdqr/1
  Fdqs/1 -> Demux/1
  Demux/2 -> Product1/1, Product2/1
  cos1/1 -> Product/2, Product2/2
  sin1/1 -> Product1/2, Product3/2
  Product/1 -> Add1/1
  Product1/1 -> Add1/2
  Add1/1 -> Mux/1
  Product2/1 -> Add2/1
  Product3/1 -> Add2/2
  Add2/1 -> Mux/2
  Gain6/1 -> sin1/1, cos1/1

== system HighFiedelity_Simulation/Mech.System/Bound PI ==
  In : Inport
  Fcn1 : Fcn  Expr=1/(2*pi)*u+0.5
  Fcn2 : Fcn  Expr=u-floor(u)
  Fcn3 : Fcn  Expr=2*pi*(u-0.5)
  Out : Outport
  wires:
  Fcn1/1 -> Fcn2/1
  Fcn2/1 -> Fcn3/1
  In/1 -> Fcn1/1
  Fcn3/1 -> Out/1

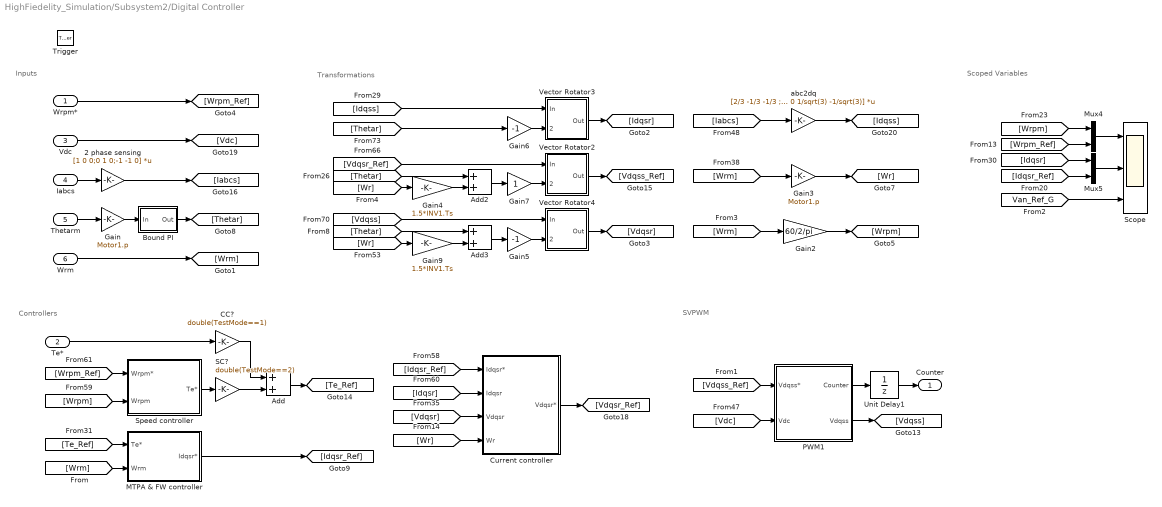
== system HighFiedelity_Simulation/Subsystem2/Digital Controller ==
  note: SVPWM
  note: Controllers
  note: Inputs
  note: Transformations
  note: Scoped Variables
  Wrpm* : Inport
  Te* : Inport  Port=2
  Vdc : Inport  Port=3
  Iabcs : Inport  Port=4
  Thetarm : Inport  Port=5
  Wrm : Inport  Port=6
  Trigger : TriggerPort  VariantControl=Variant
  2 phase sensing : Gain  Gain=[1 0 0;0 1 0;-1 -1 0]  Multiplication=Matrix(K*u)  SaturateOnIntegerOverflow=on  OutDataTypeStr=Inherit: Same as input  ParamDataTypeStr=Inherit: Same as input
  Add : Sum
  Add2 : Sum
  Add3 : Sum
  Bound PI : Subsystem
  CC? : Gain  Gain=double(TestMode==1)
  Current controller : Subsystem
  Gain : Gain  Gain=Motor1.p
  Gain2 : Gain  Gain=60/2/pi
  Gain3 : Gain  Gain=Motor1.p
  Gain4 : Gain  Gain=1.5*INV1.Ts
  Gain5 : Gain  Gain=-1
  Gain6 : Gain  Gain=-1
  Gain7 : Gain
  Gain9 : Gain  Gain=1.5*INV1.Ts
  MTPA & FW controller : Subsystem
  Mux4 : Mux  Inputs=2
  Mux5 : Mux  Inputs=2
  PWM1 : Subsystem
  SC? : Gain  Gain=double(TestMode==2)
  Scope : Scope  NumInputPorts=3
  Speed controller : Subsystem
  Unit Delay1 : UnitDelay  SampleTime=-1  HasFrameUpgradeWarning=on
  Vector Rotator2 : Subsystem
  Vector Rotator3 : Subsystem
  Vector Rotator4 : Subsystem
  abc2dq : Gain  Gain=[2/3 -1/3 -1/3 ; 0 1/sqrt(3) -1/sqrt(3)]  Multiplication=Matrix(K*u)  SaturateOnIntegerOverflow=on  OutDataTypeStr=Inherit: Same as input  ParamDataTypeStr=Inherit: Same as input
  Counter : Outport  InitialOutput=[0]
  wires:
  [Idqsr] -> Current controller/2(Idqsr)
  abc2dq/1 -> [Idqss]
  [Iabcs] -> abc2dq/1
  Vdc/1 -> [Vdc]
  [Vdqsr] -> Current controller/3(Vdqsr)
  Gain3/1 -> [Wr]
  [Wrm] -> Gain3/1
  Wrpm*/1 -> [Wrpm_Ref]
  [Idqsr_Ref] -> Current controller/1(Idqsr*)
  [Wrpm_Ref] -> Speed controller/1(Wrpm*)
  [Wrpm] -> Speed controller/2(Wrpm)
  Thetarm/1 -> Gain/1
  [Wr] -> Current controller/4(Wr)
  Gain/1 -> Bound PI/1(In)
  Bound PI/1(Out) -> [Thetar]
  Current controller/1(Vdqsr*) -> [Vdqsr_Ref]
  Unit Delay1/1 -> Counter/1
  PWM1/2(Vdqss) -> [Vdqss]
  [Vdc] -> PWM1/2(Vdc)
  [Te_Ref] -> MTPA & FW controller/1(Te*)
  CC?/1 -> Add/1
  Speed controller/1(Te*) -> SC?/1
  Add/1 -> [Te_Ref]
  Add2/1 -> Gain7/1
  Gain7/1 -> Vector Rotator2/2(Theta)
  [Vdqsr_Ref] -> Vector Rotator2/1(In)
  Vector Rotator2/1(Out) -> [Vdqss_Ref]
  [Wr] -> Gain9/1
  Gain9/1 -> Add3/2
  Add3/1 -> Gain5/1
  [Thetar] -> Add3/1
  Gain5/1 -> Vector Rotator4/2(Theta)
  [Vdqss] -> Vector Rotator4/1(In)
  Vector Rotator4/1(Out) -> [Vdqsr]
  [Vdqss_Ref] -> PWM1/1(Vdqss*)
  Gain6/1 -> Vector Rotator3/2(Theta)
  [Idqss] -> Vector Rotator3/1(In)
  Vector Rotator3/1(Out) -> [Idqsr]
  [Thetar] -> Gain6/1
  PWM1/1(Counter) -> Unit Delay1/1
  Iabcs/1 -> 2 phase sensing/1
  2 phase sensing/1 -> [Iabcs]
  MTPA & FW controller/1(Idqsr*) -> [Idqsr_Ref]
  [Wr] -> Gain4/1
  Gain4/1 -> Add2/2
  [Thetar] -> Add2/1
  [Idqsr] -> Mux5/1
  [Idqsr_Ref] -> Mux5/2
  [Wrpm] -> Mux4/1
  [Wrpm_Ref] -> Mux4/2
  SC?/1 -> Add/2
  Te*/1 -> CC?/1
  Wrm/1 -> [Wrm]
  [Wrm] -> Gain2/1
  Gain2/1 -> [Wrpm]
  Mux5/1 -> Scope/2
  [Van_Ref_G] -> Scope/3
  Mux4/1 -> Scope/1
  [Wrm] -> MTPA & FW controller/2(Wrm)

== system HighFiedelity_Simulation/Subsystem2/PWM Module ==
  Counter : Inport
  Add3 : Sum  Inputs=+-
  Relay3 : Relay  OnSwitchValue=10*eps  OffSwitchValue=-10*eps  OutDataTypeStr=double
  Repeating Sequence1 : simulink/Sources/Repeating Sequence  rep_seq_t=[0 INV1.Tsw/2 INV1.Tsw]  rep_seq_y=[0 1 0]
  Gatings : Outport
  wires:
  Add3/1 -> Relay3/1
  Relay3/1 -> Gatings/1
  Repeating Sequence1/1 -> Add3/2
  Counter/1 -> Add3/1

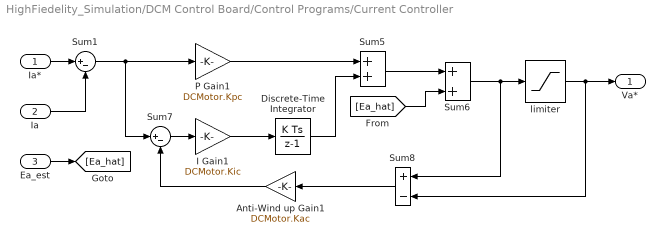
== system HighFiedelity_Simulation/DCM Control Board/Control Programs/Current Controller ==
  Ia* : Inport
  Ia : Inport  Port=2
  Ea_est : Inport  Port=3
  Anti-Wind up Gain1 : Gain  Gain=DCMotor.Kac  SaturateOnIntegerOverflow=on  OutDataTypeStr=Inherit: Same as input  ParamDataTypeStr=Inherit: Same as input
  Discrete-Time Integrator : DiscreteIntegrator  SampleTime=-1  ICPrevOutput=DiscIntNeverNeededParam  ICPrevScaledInput=DiscIntNeverNeededParam
  I Gain1 : Gain  Gain=DCMotor.Kic  SaturateOnIntegerOverflow=on  OutDataTypeStr=Inherit: Same as input  ParamDataTypeStr=Inherit: Same as input
  P Gain1 : Gain  Gain=DCMotor.Kpc  SaturateOnIntegerOverflow=on  OutDataTypeStr=Inherit: Same as input  ParamDataTypeStr=Inherit: Same as input
  Sum1 : Sum  Inputs=|+-  SaturateOnIntegerOverflow=on
  Sum5 : Sum  SaturateOnIntegerOverflow=on
  Sum6 : Sum  SaturateOnIntegerOverflow=on
  Sum7 : Sum  Inputs=|+-  SaturateOnIntegerOverflow=on
  Sum8 : Sum  Inputs=+-  SaturateOnIntegerOverflow=on
  limiter : Saturate  UpperLimit=DCMotor.Va_rated  LowerLimit=-DCMotor.Va_rated
  Va* : Outport  VectorParamsAs1DForOutWhenUnconnected=off
  wires:
  limiter/1 -> Va*/1, Sum8/2
  Sum8/1 -> Anti-Wind up Gain1/1
  Anti-Wind up Gain1/1 -> Sum7/2
  Sum7/1 -> I Gain1/1
  Sum1/1 -> Sum7/1, P Gain1/1
  P Gain1/1 -> Sum5/1
  Discrete-Time Integrator/1 -> Sum5/2
  Sum5/1 -> Sum6/1
  Sum6/1 -> limiter/1, Sum8/1
  I Gain1/1 -> Discrete-Time Integrator/1
  Ia*/1 -> Sum1/1
  [Ea_hat] -> Sum6/2
  Ia/1 -> Sum1/2
  Ea_est/1 -> [Ea_hat]

== system HighFiedelity_Simulation/DCM Control Board/Control Programs/Speed Controller ==
  note: Te*
  Wm* : Inport
  Wm : Inport  Port=2
  Discrete-Time Integrator : DiscreteIntegrator  SampleTime=-1  ICPrevOutput=DiscIntNeverNeededParam  ICPrevScaledInput=DiscIntNeverNeededParam
  Ksa : Gain  Gain=DCMotor.Ksa  SaturateOnIntegerOverflow=on  OutDataTypeStr=Inherit: Same as input  ParamDataTypeStr=Inherit: Same as input
  Ksi : Gain  Gain=DCMotor.Ksi  SaturateOnIntegerOverflow=on  OutDataTypeStr=Inherit: Same as input  ParamDataTypeStr=Inherit: Same as input
  Ksp : Gain  Gain=DCMotor.Ksp  SaturateOnIntegerOverflow=on  OutDataTypeStr=Inherit: Same as input  ParamDataTypeStr=Inherit: Same as input
  Sum : Sum  Inputs=|+-  SaturateOnIntegerOverflow=on
  Sum2 : Sum  Inputs=|+-  SaturateOnIntegerOverflow=on
  Sum3 : Sum  Inputs=++|  SaturateOnIntegerOverflow=on
  Sum4 : Sum  Inputs=+-  SaturateOnIntegerOverflow=on
  Te-limiter : Saturate  UpperLimit=DCMotor.Te_limit  LowerLimit=-DCMotor.Te_limit
  Te* : Outport  VectorParamsAs1DForOutWhenUnconnected=off
  wires:
  Ksa/1 -> Sum2/2
  Sum2/1 -> Ksi/1
  Sum4/1 -> Ksa/1
  Sum/1 -> Sum2/1, Ksp/1
  Ksi/1 -> Discrete-Time Integrator/1
  Ksp/1 -> Sum3/1
  Discrete-Time Integrator/1 -> Sum3/2
  Sum3/1 -> Sum4/1, Te-limiter/1
  Wm/1 -> Sum/2
  Te-limiter/1 -> Te*/1, Sum4/2
  Wm*/1 -> Sum/1

== system HighFiedelity_Simulation/Subsystem2/Digital Controller/Bound PI ==
  In : Inport
  Fcn1 : Fcn  Expr=1/(2*pi)*u+0.5
  Fcn2 : Fcn  Expr=u-floor(u)
  Fcn3 : Fcn  Expr=2*pi*(u-0.5)
  Out : Outport
  wires:
  Fcn1/1 -> Fcn2/1
  Fcn2/1 -> Fcn3/1
  In/1 -> Fcn1/1
  Fcn3/1 -> Out/1

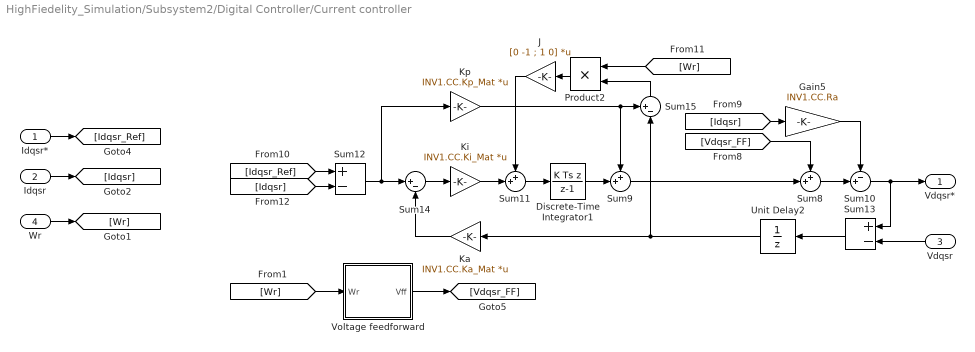
== system HighFiedelity_Simulation/Subsystem2/Digital Controller/Current controller ==
  Idqsr* : Inport
  Idqsr : Inport  Port=2
  Vdqsr : Inport  Port=3
  Wr : Inport  Port=4
  Discrete-Time Integrator1 : DiscreteIntegrator  IntegratorMethod=Integration: Backward Euler  SampleTime=-1  ICPrevOutput=DiscIntNeverNeededParam  ICPrevScaledInput=DiscIntNeverNeededParam
  Gain5 : Gain  Gain=INV1.CC.Ra
  J : Gain  Gain=[0 -1 ; 1 0]  Multiplication=Matrix(K*u)
  Ka : Gain  Gain=INV1.CC.Ka_Mat  Multiplication=Matrix(K*u)  SaturateOnIntegerOverflow=on  OutDataTypeStr=Inherit: Same as input  ParamDataTypeStr=Inherit: Same as input
  Ki : Gain  Gain=INV1.CC.Ki_Mat  Multiplication=Matrix(K*u)  SaturateOnIntegerOverflow=on  OutDataTypeStr=Inherit: Same as input  ParamDataTypeStr=Inherit: Same as input
  Kp : Gain  Gain=INV1.CC.Kp_Mat  Multiplication=Matrix(K*u)  SaturateOnIntegerOverflow=on  OutDataTypeStr=Inherit: Same as input  ParamDataTypeStr=Inherit: Same as input
  Product2 : Product  RndMeth=Zero
  Sum10 : Sum  Inputs=-+|
  Sum11 : Sum  Inputs=++|
  Sum12 : Sum  Inputs=+-
  Sum13 : Sum  Inputs=+-
  Sum14 : Sum  Inputs=|+-
  Sum15 : Sum  Inputs=+-|
  Sum8 : Sum  Inputs=++|
  Sum9 : Sum  Inputs=++|
  Unit Delay2 : UnitDelay  SampleTime=-1  HasFrameUpgradeWarning=on
  Voltage feedforward : Subsystem
  Vdqsr* : Outport
  wires:
  Idqsr/1 -> [Idqsr]
  Idqsr*/1 -> [Idqsr_Ref]
  Wr/1 -> [Wr]
  [Wr] -> Voltage feedforward/1(Wr)
  Voltage feedforward/1(Vff) -> [Vdqsr_FF]
  Discrete-Time Integrator1/1 -> Sum9/2
  Gain5/1 -> Sum10/1
  [Idqsr_Ref] -> Sum12/1
  Sum11/1 -> Discrete-Time Integrator1/1
  Ki/1 -> Sum11/2
  Kp/1 -> Sum15/1, Sum9/1
  Sum8/1 -> Sum10/2
  J/1 -> Sum11/1
  [Idqsr] -> Gain5/1
  Product2/1 -> J/1
  Sum12/1 -> Sum14/1, Kp/1
  [Idqsr] -> Sum12/2
  Sum9/1 -> Sum8/2
  [Wr] -> Product2/1
  [Vdqsr_FF] -> Sum8/1
  Sum10/1 -> Vdqsr*/1, Sum13/1
  Vdqsr/1 -> Sum13/2
  Sum13/1 -> Unit Delay2/1
  Sum14/1 -> Ki/1
  Ka/1 -> Sum14/2
  Unit Delay2/1 -> Sum15/2, Ka/1
  Sum15/1 -> Product2/2

== system HighFiedelity_Simulation/Subsystem2/Digital Controller/MTPA & FW controller ==
  Te* : Inport
  Wrm : Inport  Port=2
  MTPA : Subsystem
  Idqsr* : Outport
  wires:
  Te*/1 -> [Te_Ref]
  [Te_Ref] -> MTPA/1(Te)
  MTPA/1(Idqsr) -> [Idqsr_Ref]
  [Idqsr_Ref] -> Idqsr*/1
  Wrm/1 -> MTPA/2(Wrm)

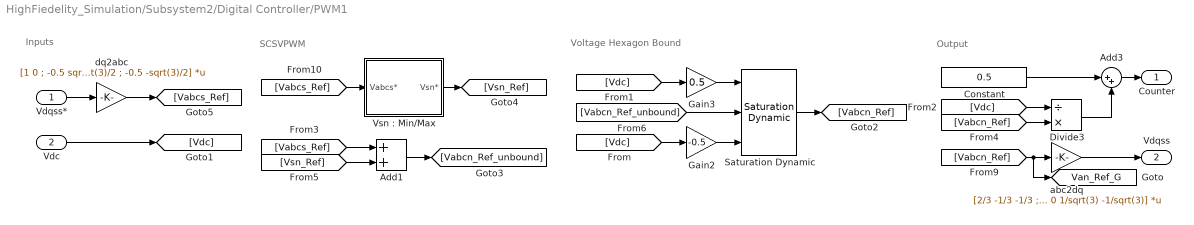
== system HighFiedelity_Simulation/Subsystem2/Digital Controller/PWM1 ==
  note: Output
  note: Voltage Hexagon Bound
  note: SCSVPWM
  note: Inputs
  Vdqss* : Inport
  Vdc : Inport  Port=2
  Add1 : Sum
  Add3 : Sum  Inputs=|++
  Constant : Constant  Value=0.5
  Divide3 : Product  Inputs=/*
  Gain2 : Gain  Gain=-0.5
  Gain3 : Gain  Gain=0.5
  Saturation Dynamic : simulink/Discontinuities/Saturation Dynamic  OutMin=[]  OutMax=[]  OutDataTypeStr=Inherit: Same as second input  OutDataType=fixdt(1, 16)  OutScaling=2^-10  DoSatur=off
  "Vsn : Min/Max" : Subsystem
  abc2dq : Gain  Gain=[2/3 -1/3 -1/3 ; 0 1/sqrt(3) -1/sqrt(3)]  Multiplication=Matrix(K*u)  SaturateOnIntegerOverflow=on  OutDataTypeStr=Inherit: Same as input  ParamDataTypeStr=Inherit: Same as input
  dq2abc : Gain  Gain=[1 0 ; -0.5 sqrt(3)/2 ; -0.5 -sqrt(3)/2]  Multiplication=Matrix(K*u)
  Counter : Outport
  Vdqss : Outport  Port=2
  tag scope: Van_Ref_G=global
  wires:
  Vdqss*/1 -> dq2abc/1
  dq2abc/1 -> [Vabcs_Ref]
  Gain2/1 -> Saturation Dynamic/3
  Vdc/1 -> [Vdc]
  Saturation Dynamic/1 -> [Vabcn_Ref]
  abc2dq/1 -> Vdqss/1
  [Vabcn_Ref] -> [Van_Ref_G], abc2dq/1
  [Vabcs_Ref] -> "Vsn : Min/Max"/1(Vabcs*)
  "Vsn : Min/Max"/1(Vsn*) -> [Vsn_Ref]
  Divide3/1 -> Add3/2
  [Vabcn_Ref] -> Divide3/2
  Constant/1 -> Add3/1
  Add3/1 -> Counter/1
  [Vdc] -> Divide3/1
  [Vabcs_Ref] -> Add1/1
  [Vsn_Ref] -> Add1/2
  Add1/1 -> [Vabcn_Ref_unbound]
  [Vdc] -> Gain2/1
  Gain3/1 -> Saturation Dynamic/1
  [Vdc] -> Gain3/1
  [Vabcn_Ref_unbound] -> Saturation Dynamic/2

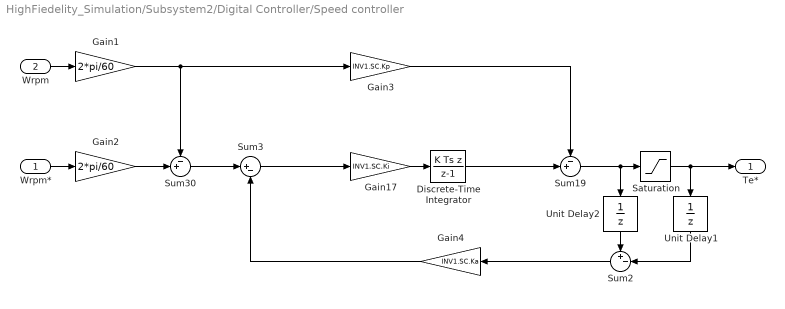
== system HighFiedelity_Simulation/Subsystem2/Digital Controller/Speed controller ==
  Wrpm* : Inport
  Wrpm : Inport  Port=2
  Discrete-Time Integrator : DiscreteIntegrator  IntegratorMethod=Integration: Backward Euler  SampleTime=-1  ICPrevOutput=DiscIntNeverNeededParam  ICPrevScaledInput=DiscIntNeverNeededParam
  Gain1 : Gain  Gain=2*pi/60
  Gain17 : Gain  Gain=INV1.SC.Ki
  Gain2 : Gain  Gain=2*pi/60
  Gain3 : Gain  Gain=INV1.SC.Kp
  Gain4 : Gain  Gain=INV1.SC.Ka
  Saturation : Saturate  UpperLimit=INV1.SC.Te_lim  LowerLimit=-INV1.SC.Te_lim
  Sum19 : Sum  Inputs=-+|
  Sum2 : Sum  Inputs=+-|
  Sum3 : Sum  Inputs=|+-
  Sum30 : Sum  Inputs=-+|
  Unit Delay1 : UnitDelay  SampleTime=-1  HasFrameUpgradeWarning=on
  Unit Delay2 : UnitDelay  SampleTime=-1  HasFrameUpgradeWarning=on
  Te* : Outport  InitialOutput=[0]
  wires:
  Gain2/1 -> Sum30/2
  Gain17/1 -> Discrete-Time Integrator/1
  Gain3/1 -> Sum19/1
  Sum3/1 -> Gain17/1
  Sum30/1 -> Sum3/1
  Unit Delay2/1 -> Sum2/1
  Gain4/1 -> Sum3/2
  Saturation/1 -> Te*/1, Unit Delay1/1
  Sum19/1 -> Saturation/1, Unit Delay2/1
  Sum2/1 -> Gain4/1
  Unit Delay1/1 -> Sum2/2
  Wrpm*/1 -> Gain2/1
  Wrpm/1 -> Gain1/1
  Discrete-Time Integrator/1 -> Sum19/2
  Gain1/1 -> Gain3/1, Sum30/1

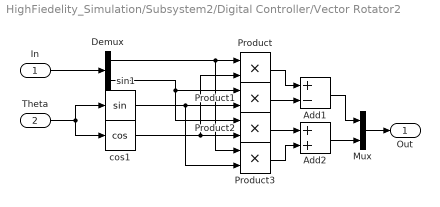
== system HighFiedelity_Simulation/Subsystem2/Digital Controller/Vector Rotator2 ==
  In : Inport
  Theta : Inport  Port=2
  Add1 : Sum  Inputs=+-
  Add2 : Sum
  Demux : Demux  Outputs=2
  Mux : Mux  Inputs=[1 1]
  Product{,1..3} (4 alike) : Product  RndMeth=Zero
  cos1 : Trigonometry  Operator=cos
  sin1 : Trigonometry
  Out : Outport
  wires:
  Theta/1 -> cos1/1, sin1/1
  Demux/1 -> Product3/1, Product/1
  Mux/1 -> Out/1
  In/1 -> Demux/1
  Demux/2 -> Product1/1, Product2/1
  cos1/1 -> Product/2, Product2/2
  sin1/1 -> Product1/2, Product3/2
  Product/1 -> Add1/1
  Product1/1 -> Add1/2
  Add1/1 -> Mux/1
  Product2/1 -> Add2/1
  Product3/1 -> Add2/2
  Add2/1 -> Mux/2

== system HighFiedelity_Simulation/Subsystem2/Digital Controller/Vector Rotator3 ==
  In : Inport
  Theta : Inport  Port=2
  Add1 : Sum  Inputs=+-
  Add2 : Sum
  Demux : Demux  Outputs=2
  Mux : Mux  Inputs=[1 1]
  Product{,1..3} (4 alike) : Product  RndMeth=Zero
  cos1 : Trigonometry  Operator=cos
  sin1 : Trigonometry
  Out : Outport
  wires:
  Theta/1 -> cos1/1, sin1/1
  Mux/1 -> Out/1
  In/1 -> Demux/1
  cos1/1 -> Product/2, Product2/2
  sin1/1 -> Product1/2, Product3/2
  Product/1 -> Add1/1
  Product1/1 -> Add1/2
  Add1/1 -> Mux/1
  Product2/1 -> Add2/1
  Product3/1 -> Add2/2
  Add2/1 -> Mux/2
  Demux/1 -> Product3/1, Product/1
  Demux/2 -> Product2/1, Product1/1

== system HighFiedelity_Simulation/Subsystem2/Digital Controller/Vector Rotator4 ==
  In : Inport
  Theta : Inport  Port=2
  Add1 : Sum  Inputs=+-
  Add2 : Sum
  Demux : Demux  Outputs=2
  Mux : Mux  Inputs=[1 1]
  Product{,1..3} (4 alike) : Product  RndMeth=Zero
  cos1 : Trigonometry  Operator=cos
  sin1 : Trigonometry
  Out : Outport
  wires:
  Add2/1 -> Mux/2
  Product3/1 -> Add2/2
  Product2/1 -> Add2/1
  Add1/1 -> Mux/1
  Product1/1 -> Add1/2
  Product/1 -> Add1/1
  sin1/1 -> Product3/2, Product1/2
  cos1/1 -> Product2/2, Product/2
  Demux/2 -> Product2/1, Product1/1
  In/1 -> Demux/1
  Mux/1 -> Out/1
  Demux/1 -> Product/1, Product3/1
  Theta/1 -> sin1/1, cos1/1

== system HighFiedelity_Simulation/Subsystem2/Digital Controller/Current controller/Voltage feedforward ==
  Wr : Inport
  Constant : Constant  Value=[INV1.Lamf_Hat;0]
  J : Gain  Gain=[0 -1 ; 1 0]  Multiplication=Matrix(K*u)
  Product : Product  RndMeth=Zero
  Vff : Outport
  wires:
  Wr/1 -> Product/2
  J/1 -> Product/1
  Product/1 -> Vff/1
  Constant/1 -> J/1

== system HighFiedelity_Simulation/Subsystem2/Digital Controller/MTPA & FW controller/MTPA ==
  Te : Inport
  Wrm : Inport  Port=2
  Gain : Gain  Gain=60/2/pi
  Mux1 : Mux  Inputs=2
  id table : Lookup_n-D  BreakpointsForDimension1=TrqTId  BreakpointsForDimension2=TrqWrId  Table=TrqIdmap  InternalRulePriority=Speed  RndMeth=Simplest  InputSameDT=on
      settings: InputPortMap=u0,u1
  iq table : Lookup_n-D  BreakpointsForDimension1=TrqTIq  BreakpointsForDimension2=TrqWrIq  Table=TrqIqmap  InternalRulePriority=Speed  RndMeth=Simplest  InputSameDT=on
      settings: InputPortMap=u0,u1
  Idqsr : Outport
  wires:
  Te/1 -> iq table/1, id table/1
  Wrm/1 -> Gain/1
  id table/1 -> Mux1/1
  iq table/1 -> Mux1/2
  Mux1/1 -> Idqsr/1
  Gain/1 -> id table/2, iq table/2

== system HighFiedelity_Simulation/Subsystem2/Digital Controller/PWM1/Vsn : Min//Max ==
  Vabcs* : Inport
  Add3 : Sum
  Gain1 : Gain  Gain=-0.5
  MinMax1 : MinMax  Function=max
  MinMax2 : MinMax
  Vsn* : Outport
  wires:
  Add3/1 -> Gain1/1
  MinMax2/1 -> Add3/2
  MinMax1/1 -> Add3/1
  [Vabcs_Ref] -> MinMax1/1, MinMax2/1
  Gain1/1 -> Vsn*/1
  Vabcs*/1 -> [Vabcs_Ref]
